simulink model "Final_Model_Project2"  (R2023b)
settings: Solver=ode4  StartTime=0.0  StopTime=1.0  FixedStep=2e-6  RelTol=1e-3
values from neighbouring files (symbols this model uses):
  abc_alphabeta = [1 (-1/2) (-1/2); 0 (sqrt(3)/2) (-sqrt(3)/2)]    [Project2.m]
  alphabeta_abc = [1 0; (-1/2) (sqrt(3)/2); (-1/2) (-sqrt(3)/2)]    [Project2.m]
  D1 = ((L_s*L_r) - ((L_m)^2))    (= 2.813723688e-07)    [Project2.m]
  f_g = 50    [Project2.m]
  init_speed_rad = ((n_minit*2*pi)/60)    (= 151.843644924)    [Project2.m]
  J = 1200    [Project2.m]
  L_m = 2.13461e-03    (= 0.00213461)    [Project2.m]
  L_r = (L_lr + L_m)    (= 0.00219953)    [Project2.m]
  L_s = (L_ls + L_m)    (= 0.00219953)    [Project2.m]
  P = 2    [Project2.m]
  R_r = 1.497e-03    (= 0.001497)    [Project2.m]
  R_s = 1.102e-03    (= 0.001102)    [Project2.m]
  V_gLL = 690    [Project2.m]
libraries: spsVoltageMeasurementLib x3, spsGroundLib x2, spsThreePhaseProgrammableVoltageSourceLib x1, sps_lib x1
settings Model: Creator=priya  LastModifiedBy=priya
settings SolverCC: AutoInsertRateTranBlk=on

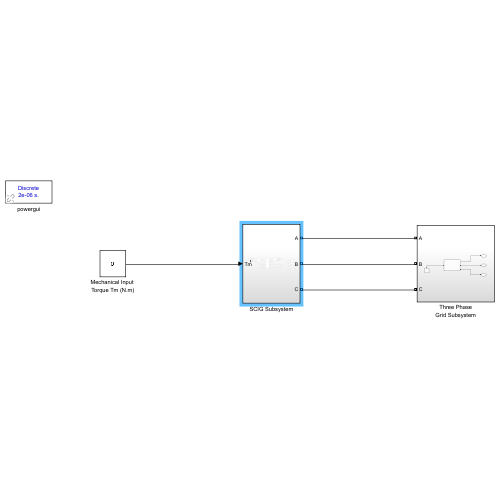
[thumbnail: Simulink's stored preview of the top-level diagram]
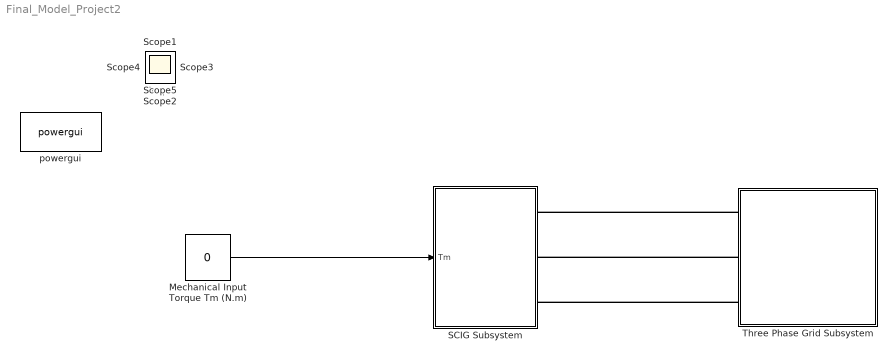
== system Final_Model_Project2 ==
  Mechanical Input Torque Tm (N.m) : Constant  Value=0
  SCIG Subsystem : Subsystem
  Three Phase Grid Subsystem : Subsystem
  powergui : sps_lib/powergui  Priority=1  SimulationMode=Discrete  SampleTime=2e-06  frequency=60  Iterations=50  frequencyindice=50  Pbase=100e6  ErrMax=1e-4  UnitsV=kV  UnitsW=MW  buscounter=0  FunctionMessages=off  echomessages=off  EnableUseOfTLC=off  CurrentSourceSwitches=off  DisableSnubberDevices=off  DisableRonSwitches=off  DisableVfSwitches=off  DisplayEquations=off  AutomaticDiscreteSolvers=off  SolverType=Tustin/Backward Euler (TBE)  Interpol=off  ExternalGateDelay=off  methode=off  Ts=100  x0status=blocks  SPID=on  SwTol=0  HookPort=off  NonlinearTolerance=1e-4  nMaxIteration=100  ContinueOnMaxIteration=off  RestoreLinks=warning  ResistiveCurrentMeasurement=off  Frange=[0:2:500]  Ylog=off  Xlog=on  ShowGrid=off  save=off  variable=ZData  structure=0  ZoomFFT=off  StartTime=0.0  cycles=1  DisplayStyle=1  fundamental=60  FreqAxis=off  MaxFrequency=1000  frequencyindicesteady=1  RmsSteady=1  display=off
  Scope{,1..5} (6 alike) : Scope
  wires:
  Mechanical Input Torque Tm (N.m)/1 -> SCIG Subsystem/1(Tm)
  connections:
  Three Phase Grid Subsystem/LConn1 -- SCIG Subsystem/RConn1
  Three Phase Grid Subsystem/LConn2 -- SCIG Subsystem/RConn2
  Three Phase Grid Subsystem/LConn3 -- SCIG Subsystem/RConn3

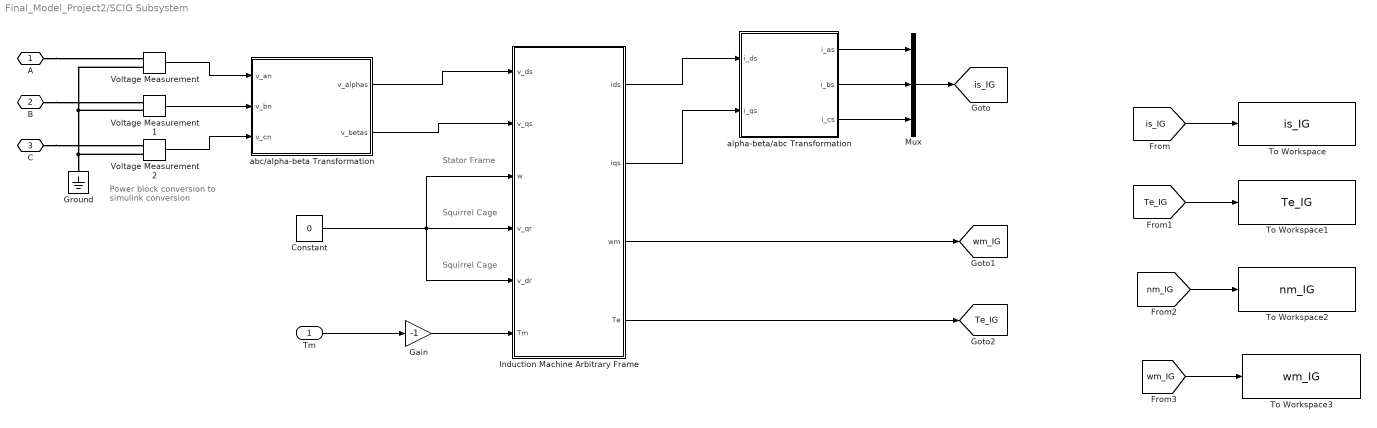
== system Final_Model_Project2/SCIG Subsystem ==
  note: Stator Frame
  note: Power block conversion
      | to simulink conversion
  note: Squirrel Cage
  note: Squirrel Cage
  Tm : Inport
  Constant : Constant  Value=0
  Gain : Gain  Gain=-1
  Ground : spsGroundLib/Ground  LConnTagsString=a
  Induction Machine Arbitrary Frame : Subsystem
  Mux : Mux  Inputs=3
  To Workspace : ToWorkspace  VariableName=is_IG  SampleTime=-1
  To Workspace1 : ToWorkspace  VariableName=Te_IG  SampleTime=-1
  To Workspace2 : ToWorkspace  VariableName=nm_IG  SampleTime=-1
  To Workspace3 : ToWorkspace  VariableName=wm_IG  SampleTime=-1
  Voltage Measurement : spsVoltageMeasurementLib/Voltage Measurement  PhasorSimulation=off  OutputType=Complex  PSBequivalent=0
  Voltage Measurement1 : spsVoltageMeasurementLib/Voltage Measurement  PhasorSimulation=off  OutputType=Complex  PSBequivalent=0
  Voltage Measurement2 : spsVoltageMeasurementLib/Voltage Measurement  PhasorSimulation=off  OutputType=Complex  PSBequivalent=0
  abc/alpha-beta Transformation : Subsystem
  alpha-beta/abc Transformation : Subsystem
  A : PMIOPort  Side=Right
  B : PMIOPort  Port=2  Side=Right
  C : PMIOPort  Port=3  Side=Right
  tag scope: Te_IG=global, is_IG=global, wm_IG=global
  wires:
  Voltage Measurement/1 -> abc/alpha-beta Transformation/1(v_an)
  Voltage Measurement1/1 -> abc/alpha-beta Transformation/2(v_bn)
  Voltage Measurement2/1 -> abc/alpha-beta Transformation/3(v_cn)
  Tm/1 -> Gain/1
  alpha-beta/abc Transformation/1(i_as) -> Mux/1
  alpha-beta/abc Transformation/2(i_bs) -> Mux/2
  alpha-beta/abc Transformation/3(i_cs) -> Mux/3
  Mux/1 -> [is_IG]
  Induction Machine Arbitrary Frame/3(wm) -> [wm_IG]
  Induction Machine Arbitrary Frame/4(Te) -> [Te_IG]
  Gain/1 -> Induction Machine Arbitrary Frame/6(Tm)
  abc/alpha-beta Transformation/2(v_betas) -> Induction Machine Arbitrary Frame/2(v_qs)
  abc/alpha-beta Transformation/1(v_alphas) -> Induction Machine Arbitrary Frame/1(v_ds)
  Constant/1 -> Induction Machine Arbitrary Frame/5(v_dr), Induction Machine Arbitrary Frame/4(v_qr), Induction Machine Arbitrary Frame/3(w)
  Induction Machine Arbitrary Frame/1(ids) -> alpha-beta/abc Transformation/1(i_ds)
  Induction Machine Arbitrary Frame/2(iqs) -> alpha-beta/abc Transformation/2(i_qs)
  [is_IG] -> To Workspace/1
  [Te_IG] -> To Workspace1/1
  [nm_IG] -> To Workspace2/1
  [wm_IG] -> To Workspace3/1
  connections:
  A/RConn1 -- Voltage Measurement/LConn1
  B/RConn1 -- Voltage Measurement1/LConn1
  C/RConn1 -- Voltage Measurement2/LConn1
  Voltage Measurement/LConn2 -- Voltage Measurement1/LConn2 -- Voltage Measurement2/LConn2 -- Ground/LConn1

== system Final_Model_Project2/Three Phase Grid Subsystem ==
  Ground1 : spsGroundLib/Ground  LConnTagsString=a
  Three-Phase Programmable Voltage Source : spsThreePhaseProgrammableVoltageSourceLib/Three-Phase Programmable Voltage Source  PositiveSequence="[V_gLL  0 f_g]"  VariationEntity=None  VariationType=Table of time-amplitude pairs  VariationTypeAlt=Step  VariationStep=0.5  VariationRate=10  VariationMagnitude=0.3  VariationFrequency=2  VariationTiming=[1 2]  VariationPhaseA=off  Amplitudes=[1 0.8 1.2 1.0]  TimeValues=[0 0.1 0.15 0.2]  HarmonicGeneration=off  HarmonicA=[3 0.2 -25 0]  HarmonicB=[2 0.15 35 2]  Timing="[0.05  3]"  BusType=swing  Pref=0  Qref=0  Qmin=-inf  Qmax=inf
  A : PMIOPort  Side=Left
  B : PMIOPort  Port=2  Side=Left
  C : PMIOPort  Port=3  Side=Left
  connections:
  Three-Phase Programmable Voltage Source/LConn1 -- Ground1/LConn1
  B/RConn1 -- Three-Phase Programmable Voltage Source/RConn2
  C/RConn1 -- Three-Phase Programmable Voltage Source/RConn3
  Three-Phase Programmable Voltage Source/RConn1 -- A/RConn1

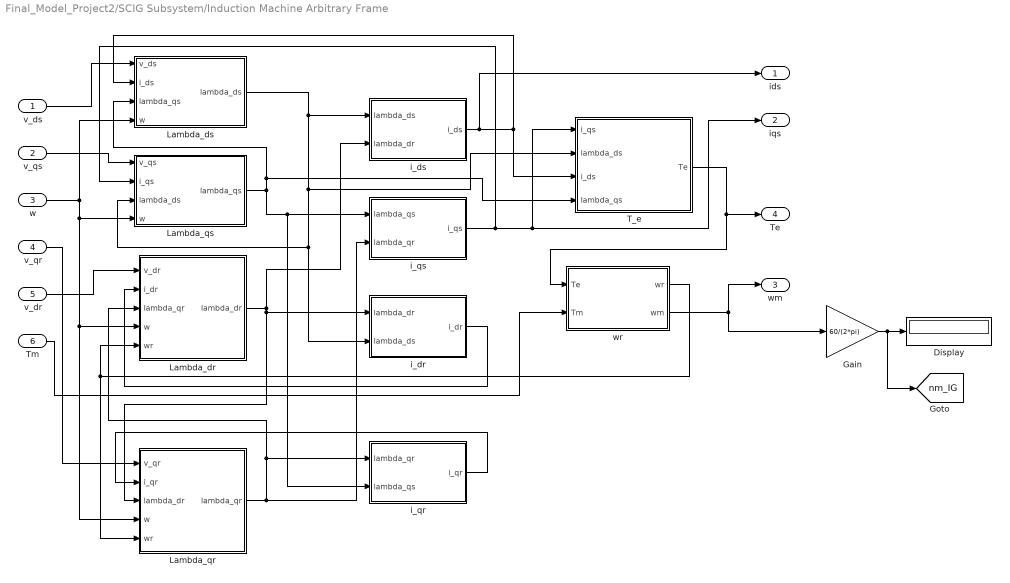
== system Final_Model_Project2/SCIG Subsystem/Induction Machine Arbitrary Frame ==
  v_ds : Inport
  v_qs : Inport  Port=2
  w : Inport  Port=3
  v_qr : Inport  Port=4
  v_dr : Inport  Port=5
  Tm : Inport  Port=6
  Display : Display
  Gain : Gain  Gain=60/(2*pi)
  Lambda_dr : Subsystem
  Lambda_ds : Subsystem
  Lambda_qr : Subsystem
  Lambda_qs : Subsystem
  T_e : Subsystem
  i_dr : Subsystem
  i_ds : Subsystem
  i_qr : Subsystem
  i_qs : Subsystem
  wr : Subsystem
  ids : Outport
  iqs : Outport  Port=2
  wm : Outport  Port=3
  Te : Outport  Port=4
  tag scope: nm_IG=global
  wires:
  v_ds/1 -> Lambda_ds/1(v_ds)
  i_ds/1(i_ds) -> ids/1, T_e/3(i_ds), Lambda_ds/2(i_ds)
  Lambda_qs/1(lambda_qs) -> i_qr/2(lambda_qs), i_qs/1(lambda_qs), Lambda_ds/3(lambda_qs), T_e/4(lambda_qs)
  w/1 -> Lambda_dr/4(w), Lambda_qr/4(w), Lambda_qs/4(w), Lambda_ds/4(w)
  Lambda_ds/1(lambda_ds) -> T_e/2(lambda_ds), i_dr/2(lambda_ds), Lambda_qs/3(lambda_ds), i_ds/1(lambda_ds)
  v_qs/1 -> Lambda_qs/1(v_qs)
  i_qs/1(i_qs) -> iqs/1, T_e/1(i_qs), Lambda_qs/2(i_qs)
  v_dr/1 -> Lambda_dr/1(v_dr)
  i_dr/1(i_dr) -> Lambda_dr/2(i_dr)
  Lambda_qr/1(lambda_qr) -> i_qs/2(lambda_qr), i_qr/1(lambda_qr), Lambda_dr/3(lambda_qr)
  wr/1(wr) -> Lambda_dr/5(wr), Lambda_qr/5(wr)
  v_qr/1 -> Lambda_qr/1(v_qr)
  i_qr/1(i_qr) -> Lambda_qr/2(i_qr)
  Lambda_dr/1(lambda_dr) -> i_dr/1(lambda_dr), Lambda_qr/3(lambda_dr), i_ds/2(lambda_dr)
  T_e/1(Te) -> wr/1(Te), Te/1
  Tm/1 -> wr/2(Tm)
  wr/2(wm) -> Gain/1, wm/1
  Gain/1 -> [nm_IG], Display/1

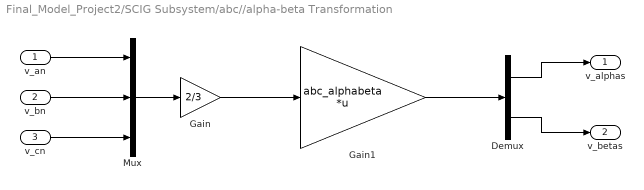
== system Final_Model_Project2/SCIG Subsystem/abc//alpha-beta Transformation ==
  v_an : Inport
  v_bn : Inport  Port=2
  v_cn : Inport  Port=3
  Demux : Demux  Outputs=2
  Gain : Gain  Gain=2/3
  Gain1 : Gain  Gain=abc_alphabeta  Multiplication=Matrix(K*u)
  Mux : Mux  Inputs=3
  v_alphas : Outport
  v_betas : Outport  Port=2
  wires:
  Demux/1 -> v_alphas/1
  Demux/2 -> v_betas/1
  v_an/1 -> Mux/1
  v_bn/1 -> Mux/2
  v_cn/1 -> Mux/3
  Mux/1 -> Gain/1
  Gain/1 -> Gain1/1
  Gain1/1 -> Demux/1

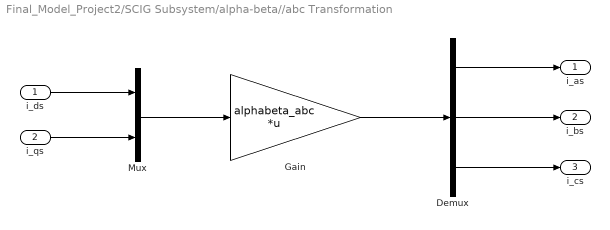
== system Final_Model_Project2/SCIG Subsystem/alpha-beta//abc Transformation ==
  i_ds : Inport
  i_qs : Inport  Port=2
  Demux : Demux  Outputs=3
  Gain : Gain  Gain=alphabeta_abc  Multiplication=Matrix(K*u)
  Mux : Mux  Inputs=2
  i_as : Outport
  i_bs : Outport  Port=2
  i_cs : Outport  Port=3
  wires:
  i_ds/1 -> Mux/1
  i_qs/1 -> Mux/2
  Demux/3 -> i_cs/1
  Demux/2 -> i_bs/1
  Demux/1 -> i_as/1
  Gain/1 -> Demux/1
  Mux/1 -> Gain/1

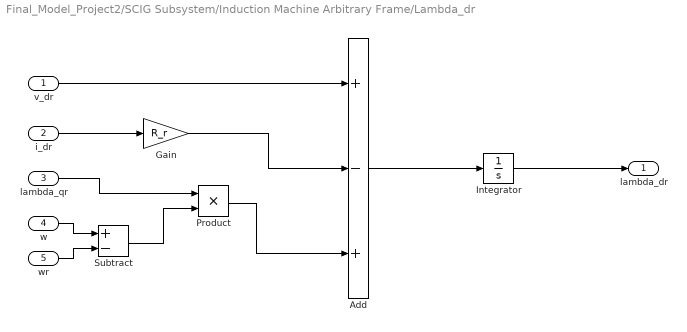
== system Final_Model_Project2/SCIG Subsystem/Induction Machine Arbitrary Frame/Lambda_dr ==
  v_dr : Inport
  i_dr : Inport  Port=2
  lambda_qr : Inport  Port=3
  w : Inport  Port=4
  wr : Inport  Port=5
  Add : Sum  Inputs=+-+
  Gain : Gain  Gain=R_r
  Integrator : Integrator
  Product : Product
  Subtract : Sum  Inputs=+-
  lambda_dr : Outport
  wires:
  Subtract/1 -> Product/2
  wr/1 -> Subtract/2
  w/1 -> Subtract/1
  Integrator/1 -> lambda_dr/1
  Add/1 -> Integrator/1
  Product/1 -> Add/3
  lambda_qr/1 -> Product/1
  Gain/1 -> Add/2
  i_dr/1 -> Gain/1
  v_dr/1 -> Add/1

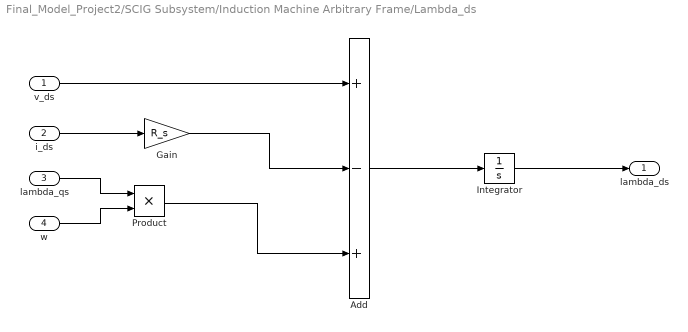
== system Final_Model_Project2/SCIG Subsystem/Induction Machine Arbitrary Frame/Lambda_ds ==
  v_ds : Inport
  i_ds : Inport  Port=2
  lambda_qs : Inport  Port=3
  w : Inport  Port=4
  Add : Sum  Inputs=+-+
  Gain : Gain  Gain=R_s
  Integrator : Integrator
  Product : Product
  lambda_ds : Outport
  wires:
  v_ds/1 -> Add/1
  i_ds/1 -> Gain/1
  Gain/1 -> Add/2
  lambda_qs/1 -> Product/1
  w/1 -> Product/2
  Product/1 -> Add/3
  Add/1 -> Integrator/1
  Integrator/1 -> lambda_ds/1

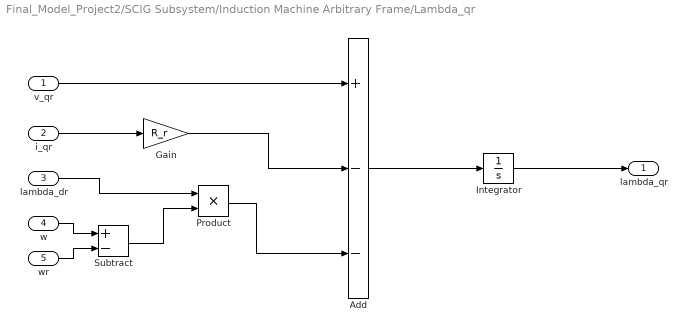
== system Final_Model_Project2/SCIG Subsystem/Induction Machine Arbitrary Frame/Lambda_qr ==
  v_qr : Inport
  i_qr : Inport  Port=2
  lambda_dr : Inport  Port=3
  w : Inport  Port=4
  wr : Inport  Port=5
  Add : Sum  Inputs=+--
  Gain : Gain  Gain=R_r
  Integrator : Integrator
  Product : Product
  Subtract : Sum  Inputs=+-
  lambda_qr : Outport
  wires:
  v_qr/1 -> Add/1
  i_qr/1 -> Gain/1
  Gain/1 -> Add/2
  lambda_dr/1 -> Product/1
  Product/1 -> Add/3
  Add/1 -> Integrator/1
  Integrator/1 -> lambda_qr/1
  w/1 -> Subtract/1
  wr/1 -> Subtract/2
  Subtract/1 -> Product/2

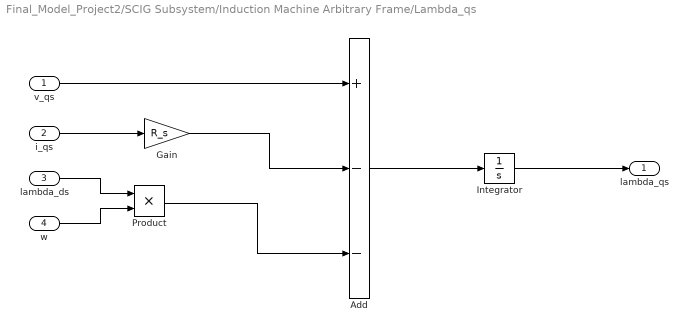
== system Final_Model_Project2/SCIG Subsystem/Induction Machine Arbitrary Frame/Lambda_qs ==
  v_qs : Inport
  i_qs : Inport  Port=2
  lambda_ds : Inport  Port=3
  w : Inport  Port=4
  Add : Sum  Inputs=+--
  Gain : Gain  Gain=R_s
  Integrator : Integrator
  Product : Product
  lambda_qs : Outport
  wires:
  Integrator/1 -> lambda_qs/1
  Add/1 -> Integrator/1
  Product/1 -> Add/3
  w/1 -> Product/2
  lambda_ds/1 -> Product/1
  Gain/1 -> Add/2
  i_qs/1 -> Gain/1
  v_qs/1 -> Add/1

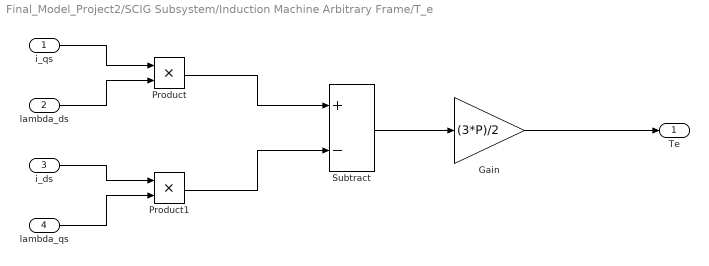
== system Final_Model_Project2/SCIG Subsystem/Induction Machine Arbitrary Frame/T_e ==
  i_qs : Inport
  lambda_ds : Inport  Port=2
  i_ds : Inport  Port=3
  lambda_qs : Inport  Port=4
  Gain : Gain  Gain=(3*P)/2
  Product : Product
  Product1 : Product
  Subtract : Sum  Inputs=+-
  Te : Outport
  wires:
  i_qs/1 -> Product/1
  lambda_ds/1 -> Product/2
  i_ds/1 -> Product1/1
  lambda_qs/1 -> Product1/2
  Product/1 -> Subtract/1
  Product1/1 -> Subtract/2
  Subtract/1 -> Gain/1
  Gain/1 -> Te/1

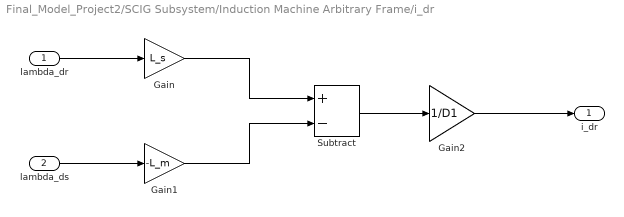
== system Final_Model_Project2/SCIG Subsystem/Induction Machine Arbitrary Frame/i_dr ==
  lambda_dr : Inport
  lambda_ds : Inport  Port=2
  Gain : Gain  Gain=L_s
  Gain1 : Gain  Gain=-L_m
  Gain2 : Gain  Gain=1/D1
  Subtract : Sum  Inputs=+-
  i_dr : Outport
  wires:
  lambda_dr/1 -> Gain/1
  Gain/1 -> Subtract/1
  lambda_ds/1 -> Gain1/1
  Gain1/1 -> Subtract/2
  Subtract/1 -> Gain2/1
  Gain2/1 -> i_dr/1

== system Final_Model_Project2/SCIG Subsystem/Induction Machine Arbitrary Frame/i_ds ==
  lambda_ds : Inport
  lambda_dr : Inport  Port=2
  Gain : Gain  Gain=L_r
  Gain1 : Gain  Gain=-L_m
  Gain2 : Gain  Gain=1/D1
  Subtract : Sum  Inputs=+-
  i_ds : Outport
  wires:
  lambda_ds/1 -> Gain/1
  Gain/1 -> Subtract/1
  lambda_dr/1 -> Gain1/1
  Gain1/1 -> Subtract/2
  Subtract/1 -> Gain2/1
  Gain2/1 -> i_ds/1

== system Final_Model_Project2/SCIG Subsystem/Induction Machine Arbitrary Frame/i_qr ==
  lambda_qr : Inport
  lambda_qs : Inport  Port=2
  Gain : Gain  Gain=L_s
  Gain1 : Gain  Gain=-L_m
  Gain2 : Gain  Gain=1/D1
  Subtract : Sum  Inputs=+-
  i_qr : Outport
  wires:
  Gain2/1 -> i_qr/1
  Subtract/1 -> Gain2/1
  Gain1/1 -> Subtract/2
  lambda_qs/1 -> Gain1/1
  Gain/1 -> Subtract/1
  lambda_qr/1 -> Gain/1

== system Final_Model_Project2/SCIG Subsystem/Induction Machine Arbitrary Frame/i_qs ==
  lambda_qs : Inport
  lambda_qr : Inport  Port=2
  Gain : Gain  Gain=L_r
  Gain1 : Gain  Gain=-L_m
  Gain2 : Gain  Gain=1/D1
  Subtract : Sum  Inputs=+-
  i_qs : Outport
  wires:
  Gain2/1 -> i_qs/1
  Subtract/1 -> Gain2/1
  Gain1/1 -> Subtract/2
  lambda_qr/1 -> Gain1/1
  Gain/1 -> Subtract/1
  lambda_qs/1 -> Gain/1

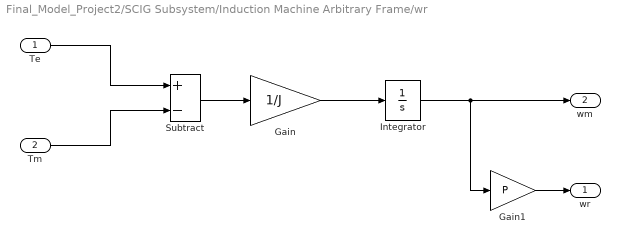
== system Final_Model_Project2/SCIG Subsystem/Induction Machine Arbitrary Frame/wr ==
  Te : Inport
  Tm : Inport  Port=2
  Gain : Gain  Gain=1/J
  Gain1 : Gain  Gain=P
  Integrator : Integrator  InitialCondition=init_speed_rad
  Subtract : Sum  Inputs=+-
  wr : Outport
  wm : Outport  Port=2
  wires:
  Te/1 -> Subtract/1
  Tm/1 -> Subtract/2
  Subtract/1 -> Gain/1
  Gain/1 -> Integrator/1
  Integrator/1 -> wm/1, Gain1/1
  Gain1/1 -> wr/1
